simulink model "TST_OilT_DD"  (R2016b)
settings: Solver=FixedStepDiscrete  StartTime=0.0  StopTime=simTime  FixedStep=sampleTime  RelTol=1e-3
values from neighbouring files (symbols this model uses):
  testCase = 1    [initTST_OilT_DD_001.m]
libraries: simulink x2
settings Model: Creator=wolf072601  LastModifiedBy=wolf072601
settings DebuggingCC: SignalRangeChecking=error
settings ConfigComp: CovEnable=on  RecordCoverage=on  CovFilter=E:\T4_WOLFFU\build\UnitTest\OilT_DD\slcov_output\OilT_DD_covfilter.cvf  CovHTMLOptions=-sRT=0  CovHtmlReporting=on  CovSaveCumulativeToWorkspaceVar=on  CovCumulativeVarName=OilT_DD_covCumulativeData  CovCumulativeReport=on  CovShowResultsExplorer=off  CovModelRefEnable=on

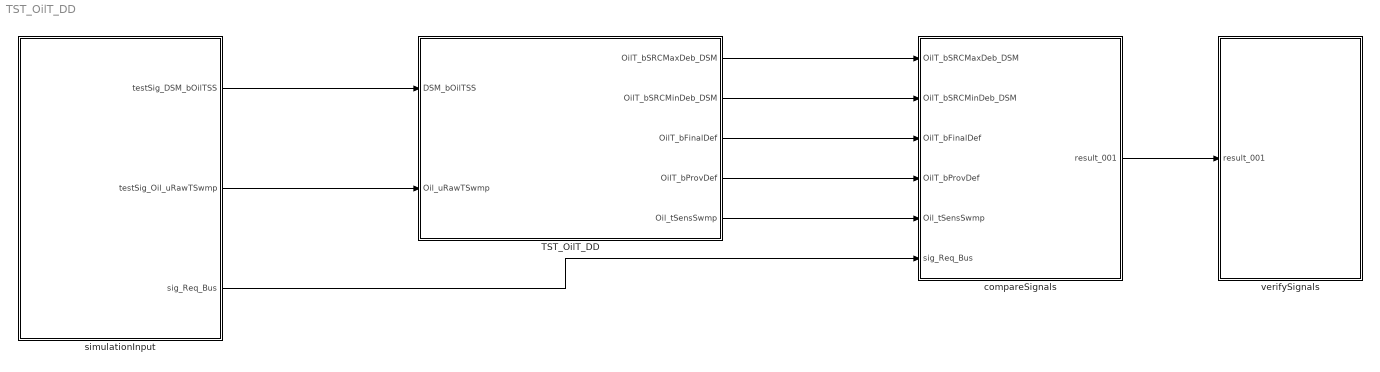
== system TST_OilT_DD ==
  TST_OilT_DD : Subsystem
  compareSignals : Subsystem
  simulationInput : Subsystem
  verifySignals : Subsystem
  wires:
  simulationInput/1(testSig_DSM_bOilTSS) -> TST_OilT_DD/1(DSM_bOilTSS)
  simulationInput/2(testSig_Oil_uRawTSwmp) -> TST_OilT_DD/2(Oil_uRawTSwmp)
  TST_OilT_DD/1(OilT_bSRCMaxDeb_DSM) -> compareSignals/1(OilT_bSRCMaxDeb_DSM)
  TST_OilT_DD/2(OilT_bSRCMinDeb_DSM) -> compareSignals/2(OilT_bSRCMinDeb_DSM)
  TST_OilT_DD/3(OilT_bFinalDef) -> compareSignals/3(OilT_bFinalDef)
  TST_OilT_DD/4(OilT_bProvDef) -> compareSignals/4(OilT_bProvDef)
  TST_OilT_DD/5(Oil_tSensSwmp) -> compareSignals/5(Oil_tSensSwmp)
  simulationInput/3(sig_Req_Bus) -> compareSignals/6(sig_Req_Bus)
  compareSignals/1(result_001) -> verifySignals/1(result_001)

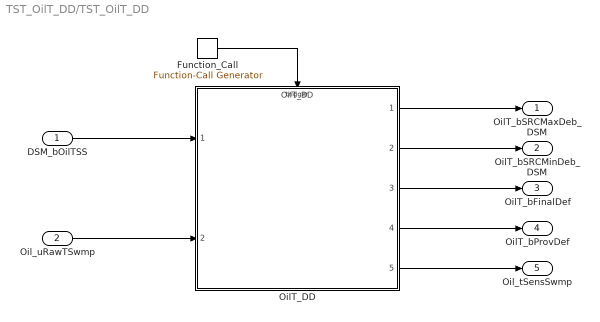
== system TST_OilT_DD/TST_OilT_DD ==
  DSM_bOilTSS : Inport
  Oil_uRawTSwmp : Inport  Port=2
  Function_Call : simulink/Ports & Subsystems/Function-Call Generator  sample_time=sampleTime  numberOfIterations=1
  OilT_DD : ModelReference  ModelNameDialog=OilT_DD  SimulationMode=Normal  ModelReferenceVersion=1.2  TriggerPortName=function  TriggerPortTriggerType=function-call  TriggerPortStatesWhenEnabling=held
  OilT_bSRCMaxDeb_DSM : Outport
  OilT_bSRCMinDeb_DSM : Outport  Port=2
  OilT_bFinalDef : Outport  Port=3
  OilT_bProvDef : Outport  Port=4
  Oil_tSensSwmp : Outport  Port=5
  wires:
  Function_Call/1 -> OilT_DD/Trigger
  DSM_bOilTSS/1 -> OilT_DD/1
  Oil_uRawTSwmp/1 -> OilT_DD/2
  OilT_DD/1 -> OilT_bSRCMaxDeb_DSM/1
  OilT_DD/2 -> OilT_bSRCMinDeb_DSM/1
  OilT_DD/3 -> OilT_bFinalDef/1
  OilT_DD/4 -> OilT_bProvDef/1
  OilT_DD/5 -> Oil_tSensSwmp/1

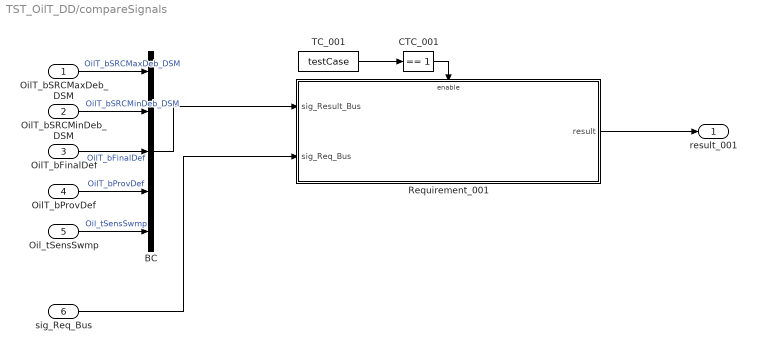
== system TST_OilT_DD/compareSignals ==
  OilT_bSRCMaxDeb_DSM : Inport
  OilT_bSRCMinDeb_DSM : Inport  Port=2
  OilT_bFinalDef : Inport  Port=3
  OilT_bProvDef : Inport  Port=4
  Oil_tSensSwmp : Inport  Port=5
  sig_Req_Bus : Inport  Port=6
  BC : BusCreator  Inputs=5
  CTC_001 : simulink/Logic and Bit Operations/Compare To Constant  relop===  const=1  OutDataTypeStr=boolean
  Requirement_001 : Subsystem
  TC_001 : Constant  Value=testCase
  result_001 : Outport
  wires:
  OilT_bSRCMaxDeb_DSM/1 -> BC/1  "OilT_bSRCMaxDeb_DSM"
  OilT_bSRCMinDeb_DSM/1 -> BC/2  "OilT_bSRCMinDeb_DSM"
  OilT_bFinalDef/1 -> BC/3  "OilT_bFinalDef"
  OilT_bProvDef/1 -> BC/4  "OilT_bProvDef"
  Oil_tSensSwmp/1 -> BC/5  "Oil_tSensSwmp"
  TC_001/1 -> CTC_001/1
  CTC_001/1 -> Requirement_001/Enable
  sig_Req_Bus/1 -> Requirement_001/2(sig_Req_Bus)
  BC/1 -> Requirement_001/1(sig_Result_Bus)
  Requirement_001/1(result) -> result_001/1

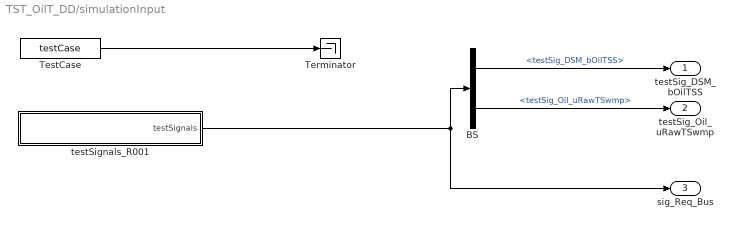
== system TST_OilT_DD/simulationInput ==
  BS : BusSelector  OutputSignals=testSig_DSM_bOilTSS,testSig_Oil_uRawTSwmp
  Terminator : Terminator
  TestCase : Constant  Value=testCase
  testSignals_R001 : Subsystem
  testSig_DSM_bOilTSS : Outport
  testSig_Oil_uRawTSwmp : Outport  Port=2
  sig_Req_Bus : Outport  Port=3
  wires:
  BS/1 -> testSig_DSM_bOilTSS/1  "<testSig_DSM_bOilTSS>"
  BS/2 -> testSig_Oil_uRawTSwmp/1  "<testSig_Oil_uRawTSwmp>"
  testSignals_R001/1(testSignals) -> BS/1, sig_Req_Bus/1
  TestCase/1 -> Terminator/1

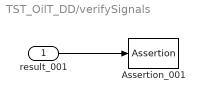
== system TST_OilT_DD/verifySignals ==
  result_001 : Inport
  Assertion_001 : Assertion
  wires:
  result_001/1 -> Assertion_001/1

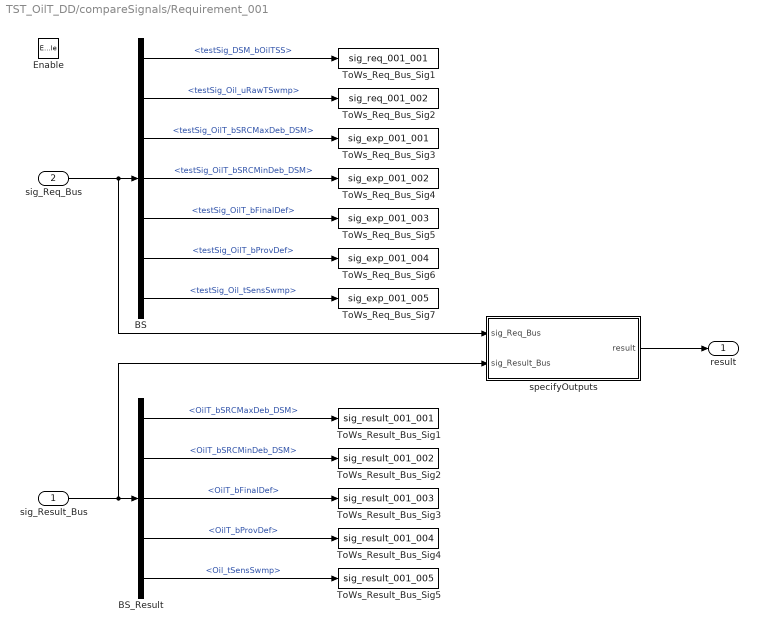
== system TST_OilT_DD/compareSignals/Requirement_001 ==
  sig_Result_Bus : Inport
  sig_Req_Bus : Inport  Port=2
  Enable : EnablePort
  BS : BusSelector  OutputSignals=testSig_DSM_bOilTSS,testSig_Oil_uRawTSwmp,testSig_OilT_bSRCMaxDeb_DSM,testSig_OilT_bSRCMinDeb_DSM,testSig_OilT_bFinalDef,testSig_OilT_bProvDef,testSig_Oil_tSensSwmp
  BS_Result : BusSelector  OutputSignals=OilT_bSRCMaxDeb_DSM,OilT_bSRCMinDeb_DSM,OilT_bFinalDef,OilT_bProvDef,Oil_tSensSwmp
  ToWs_Req_Bus_Sig1 : ToWorkspace  VariableName=sig_req_001_001  SaveFormat=Structure With Time
  ToWs_Req_Bus_Sig2 : ToWorkspace  VariableName=sig_req_001_002  SaveFormat=Structure With Time
  ToWs_Req_Bus_Sig3 : ToWorkspace  VariableName=sig_exp_001_001  SaveFormat=Structure With Time
  ToWs_Req_Bus_Sig4 : ToWorkspace  VariableName=sig_exp_001_002  SaveFormat=Structure With Time
  ToWs_Req_Bus_Sig5 : ToWorkspace  VariableName=sig_exp_001_003  SaveFormat=Structure With Time
  ToWs_Req_Bus_Sig6 : ToWorkspace  VariableName=sig_exp_001_004  SaveFormat=Structure With Time
  ToWs_Req_Bus_Sig7 : ToWorkspace  VariableName=sig_exp_001_005  SaveFormat=Structure With Time
  ToWs_Result_Bus_Sig1 : ToWorkspace  VariableName=sig_result_001_001  SaveFormat=Structure With Time
  ToWs_Result_Bus_Sig2 : ToWorkspace  VariableName=sig_result_001_002  SaveFormat=Structure With Time
  ToWs_Result_Bus_Sig3 : ToWorkspace  VariableName=sig_result_001_003  SaveFormat=Structure With Time
  ToWs_Result_Bus_Sig4 : ToWorkspace  VariableName=sig_result_001_004  SaveFormat=Structure With Time
  ToWs_Result_Bus_Sig5 : ToWorkspace  VariableName=sig_result_001_005  SaveFormat=Structure With Time
  specifyOutputs : Subsystem
  result : Outport
  wires:
  sig_Req_Bus/1 -> BS/1, specifyOutputs/1(sig_Req_Bus)
  BS/1 -> ToWs_Req_Bus_Sig1/1  "<testSig_DSM_bOilTSS>"
  BS/2 -> ToWs_Req_Bus_Sig2/1  "<testSig_Oil_uRawTSwmp>"
  BS/3 -> ToWs_Req_Bus_Sig3/1  "<testSig_OilT_bSRCMaxDeb_DSM>"
  BS/4 -> ToWs_Req_Bus_Sig4/1  "<testSig_OilT_bSRCMinDeb_DSM>"
  BS/5 -> ToWs_Req_Bus_Sig5/1  "<testSig_OilT_bFinalDef>"
  BS/6 -> ToWs_Req_Bus_Sig6/1  "<testSig_OilT_bProvDef>"
  BS/7 -> ToWs_Req_Bus_Sig7/1  "<testSig_Oil_tSensSwmp>"
  sig_Result_Bus/1 -> BS_Result/1, specifyOutputs/2(sig_Result_Bus)
  BS_Result/1 -> ToWs_Result_Bus_Sig1/1  "<OilT_bSRCMaxDeb_DSM>"
  BS_Result/2 -> ToWs_Result_Bus_Sig2/1  "<OilT_bSRCMinDeb_DSM>"
  BS_Result/3 -> ToWs_Result_Bus_Sig3/1  "<OilT_bFinalDef>"
  BS_Result/4 -> ToWs_Result_Bus_Sig4/1  "<OilT_bProvDef>"
  BS_Result/5 -> ToWs_Result_Bus_Sig5/1  "<Oil_tSensSwmp>"
  specifyOutputs/1(result) -> result/1

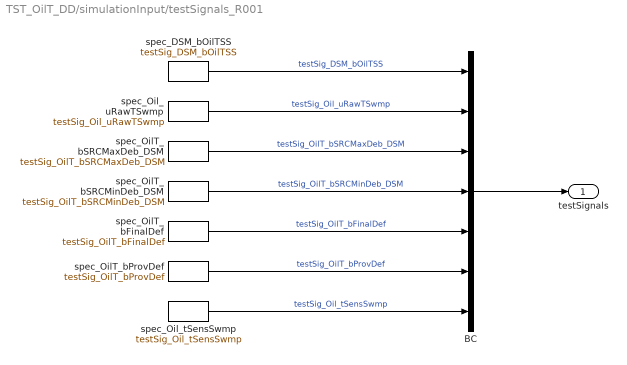
== system TST_OilT_DD/simulationInput/testSignals_R001 ==
  BC : BusCreator  Inputs=7
  spec_DSM_bOilTSS : FromWorkspace  VariableName=testSig_DSM_bOilTSS  Interpolate=off  OutputAfterFinalValue=Holding final value
  spec_OilT_bFinalDef : FromWorkspace  VariableName=testSig_OilT_bFinalDef  Interpolate=off  OutputAfterFinalValue=Holding final value
  spec_OilT_bProvDef : FromWorkspace  VariableName=testSig_OilT_bProvDef  Interpolate=off  OutputAfterFinalValue=Holding final value
  spec_OilT_bSRCMaxDeb_DSM : FromWorkspace  VariableName=testSig_OilT_bSRCMaxDeb_DSM  Interpolate=off  OutputAfterFinalValue=Holding final value
  spec_OilT_bSRCMinDeb_DSM : FromWorkspace  VariableName=testSig_OilT_bSRCMinDeb_DSM  Interpolate=off  OutputAfterFinalValue=Holding final value
  spec_Oil_tSensSwmp : FromWorkspace  VariableName=testSig_Oil_tSensSwmp  Interpolate=off  OutputAfterFinalValue=Holding final value
  spec_Oil_uRawTSwmp : FromWorkspace  VariableName=testSig_Oil_uRawTSwmp  Interpolate=off  OutputAfterFinalValue=Holding final value
  testSignals : Outport
  wires:
  BC/1 -> testSignals/1
  spec_DSM_bOilTSS/1 -> BC/1  "testSig_DSM_bOilTSS"
  spec_Oil_uRawTSwmp/1 -> BC/2  "testSig_Oil_uRawTSwmp"
  spec_OilT_bSRCMaxDeb_DSM/1 -> BC/3  "testSig_OilT_bSRCMaxDeb_DSM"
  spec_OilT_bSRCMinDeb_DSM/1 -> BC/4  "testSig_OilT_bSRCMinDeb_DSM"
  spec_OilT_bFinalDef/1 -> BC/5  "testSig_OilT_bFinalDef"
  spec_OilT_bProvDef/1 -> BC/6  "testSig_OilT_bProvDef"
  spec_Oil_tSensSwmp/1 -> BC/7  "testSig_Oil_tSensSwmp"

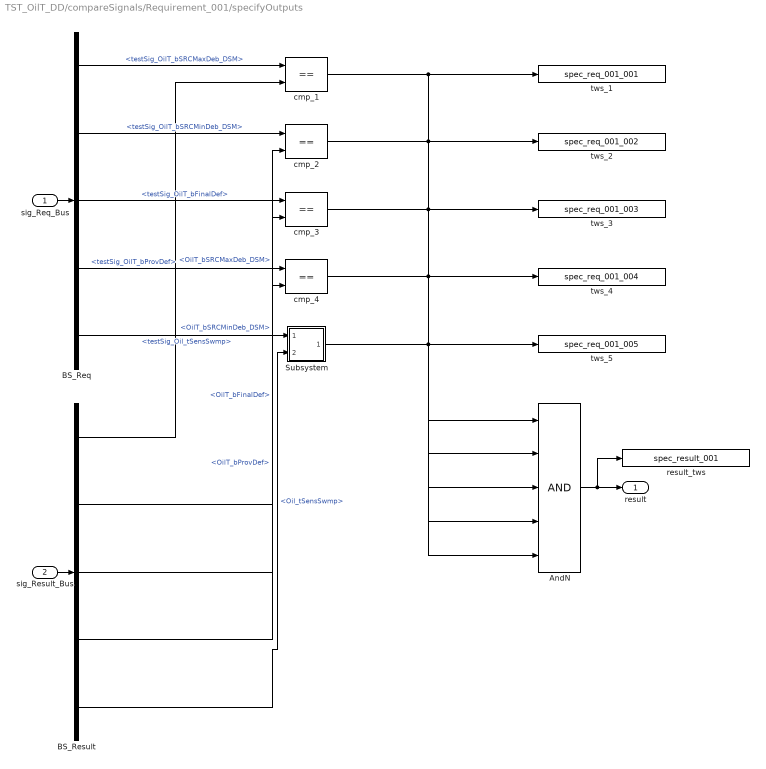
== system TST_OilT_DD/compareSignals/Requirement_001/specifyOutputs ==
  sig_Req_Bus : Inport
  sig_Result_Bus : Inport  Port=2
  AndN : Logic  Inputs=5
  BS_Req : BusSelector  OutputSignals=testSig_OilT_bSRCMaxDeb_DSM,testSig_OilT_bSRCMinDeb_DSM,testSig_OilT_bFinalDef,testSig_OilT_bProvDef,testSig_Oil_tSensSwmp
  BS_Result : BusSelector  OutputSignals=OilT_bSRCMaxDeb_DSM,OilT_bSRCMinDeb_DSM,OilT_bFinalDef,OilT_bProvDef,Oil_tSensSwmp
  Subsystem : Subsystem
  cmp_{1..4} (4 alike) : RelationalOperator  Operator===  RndMeth=Nearest  InputSameDT=on
  result_tws : ToWorkspace  VariableName=spec_result_001
  tws_1 : ToWorkspace  VariableName=spec_req_001_001
  tws_2 : ToWorkspace  VariableName=spec_req_001_002
  tws_3 : ToWorkspace  VariableName=spec_req_001_003
  tws_4 : ToWorkspace  VariableName=spec_req_001_004
  tws_5 : ToWorkspace  VariableName=spec_req_001_005
  result : Outport
  wires:
  sig_Req_Bus/1 -> BS_Req/1
  sig_Result_Bus/1 -> BS_Result/1
  AndN/1 -> result/1, result_tws/1
  BS_Req/1 -> cmp_1/1  "<testSig_OilT_bSRCMaxDeb_DSM>"
  BS_Result/1 -> cmp_1/2  "<OilT_bSRCMaxDeb_DSM>"
  cmp_1/1 -> tws_1/1, AndN/1
  BS_Req/2 -> cmp_2/1  "<testSig_OilT_bSRCMinDeb_DSM>"
  BS_Result/2 -> cmp_2/2  "<OilT_bSRCMinDeb_DSM>"
  cmp_2/1 -> tws_2/1, AndN/2
  BS_Req/3 -> cmp_3/1  "<testSig_OilT_bFinalDef>"
  BS_Result/3 -> cmp_3/2  "<OilT_bFinalDef>"
  cmp_3/1 -> tws_3/1, AndN/3
  BS_Req/4 -> cmp_4/1  "<testSig_OilT_bProvDef>"
  BS_Result/4 -> cmp_4/2  "<OilT_bProvDef>"
  cmp_4/1 -> tws_4/1, AndN/4
  BS_Req/5 -> Subsystem/1(In1)  "<testSig_Oil_tSensSwmp>"
  BS_Result/5 -> Subsystem/2(In2)  "<Oil_tSensSwmp>"
  Subsystem/1(Out1) -> tws_5/1, AndN/5

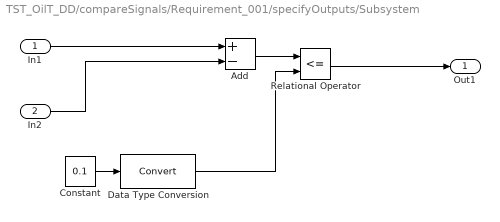
== system TST_OilT_DD/compareSignals/Requirement_001/specifyOutputs/Subsystem ==
  In1 : Inport
  In2 : Inport  Port=2
  Add : Sum  Inputs=+-
  Constant : Constant  Value=0.1
  Data Type Conversion : DataTypeConversion
  Relational Operator : RelationalOperator  Operator=<=  OutDataTypeStr=boolean  RndMeth=Simplest
  Out1 : Outport
  wires:
  In1/1 -> Add/1
  In2/1 -> Add/2
  Constant/1 -> Data Type Conversion/1
  Add/1 -> Relational Operator/1
  Data Type Conversion/1 -> Relational Operator/2
  Relational Operator/1 -> Out1/1
